simulink model "LOTS_2023_sim"  (R2022a)
settings: Solver=VariableStepAuto  StartTime=0.0  StopTime=10.0  RelTol=1e-3
model workspace (MAT data in the model file):
  v_burnout = 0
undefined symbols (not defined in the file or in its folder): or_Cd_const
libraries: aerolibatmos2 x1
settings Model: Creator=joedo  LastModifiedBy=joedo

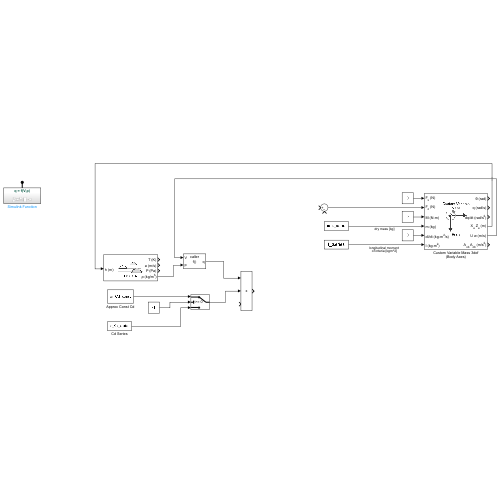
[thumbnail: Simulink's stored preview of the top-level diagram]
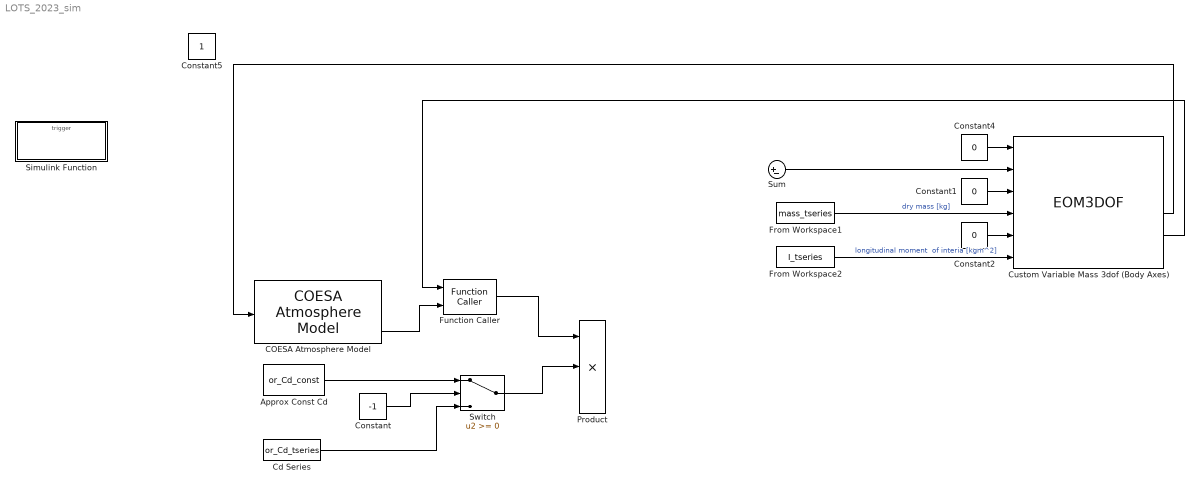
== system LOTS_2023_sim ==
  Approx Const Cd : Constant  Value=or_Cd_const
  COESA Atmosphere Model : aerolibatmos2/COESA Atmosphere Model  units=Metric (MKS)  spec=1976 COESA-extended U.S. Standard Atmosphere  model=Profile  profile_var=High temperature  profile_percent=1%  profile_alt=5 km (16404 ft)  envelope_var=High temperature  envelope_percent=1%  action=Warning
  Cd Series : FromWorkspace  VariableName=or_Cd_tseries
  Constant : Constant  Value=-1
  Constant1 : Constant  Value=0
  Constant2 : Constant  Value=0
  Constant4 : Constant  Value=0
  Custom Variable Mass 3dof (Body Axes) : EOM3DOF  mtype=Custom Variable  v_ini=v_burnout
  From Workspace1 : FromWorkspace  VariableName=mass_tseries
  From Workspace2 : FromWorkspace  VariableName=I_tseries
  Function Caller : FunctionCaller  FunctionPrototype=q = f(V,p)  InputArgumentSpecifications=<Enter example>  OutputArgumentSpecifications=<Enter example>
  Product : Product  Inputs=3
  Simulink Function : Subsystem  TreatAsAtomicUnit=on
  Sum : Sum  Inputs=|+-
  Switch : Switch  SaturateOnIntegerOverflow=off  InputSameDT=off
  Constant5 : Constant  IOType=siggen
  wires:
  From Workspace1/1 -> Custom Variable Mass 3dof (Body Axes)/4  "dry mass [kg]"
  Constant1/1 -> Custom Variable Mass 3dof (Body Axes)/3
  Constant2/1 -> Custom Variable Mass 3dof (Body Axes)/5
  Constant4/1 -> Custom Variable Mass 3dof (Body Axes)/1
  From Workspace2/1 -> Custom Variable Mass 3dof (Body Axes)/6  "longitudinal moment  of interia [kgm^2]"
  Sum/1 -> Custom Variable Mass 3dof (Body Axes)/2
  Custom Variable Mass 3dof (Body Axes)/4 -> COESA Atmosphere Model/1
  Custom Variable Mass 3dof (Body Axes)/5 -> Function Caller/1
  COESA Atmosphere Model/4 -> Function Caller/2
  Function Caller/1 -> Product/1
  Switch/1 -> Product/2
  Approx Const Cd/1 -> Switch/1
  Constant/1 -> Switch/2
  Cd Series/1 -> Switch/3

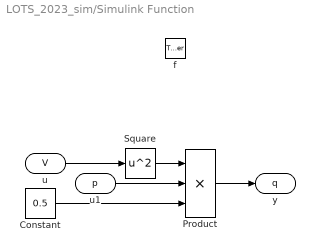
== system LOTS_2023_sim/Simulink Function ==
  f : TriggerPort  TriggerType=function-call  IsSimulinkFunction=on  FunctionName=f  FunctionVisibility=scoped  VariantControl=(inherit)
  Constant : Constant  Value=0.5
  Product : Product  Inputs=3
  Square : Math  Operator=square
  u : ArgIn  DisableCoverage=on  ArgumentName=V
  u1 : ArgIn  DisableCoverage=on  Port=2  ArgumentName=p
  y : ArgOut  DisableCoverage=on  ArgumentName=q
  wires:
  Product/1 -> y/1
  u1/1 -> Product/2
  u/1 -> Square/1
  Square/1 -> Product/1
  Constant/1 -> Product/3
